simulink model "chap6_6sim"  (Simulink 6.3)
settings: Solver=ode45  StartTime=0.0  StopTime=10  FixedStep=0.001  RelTol=1e-3
settings Model: Creator=hp  LastModifiedBy=Administrator
settings DebuggingCC: SolverPrmCheckMsg=none

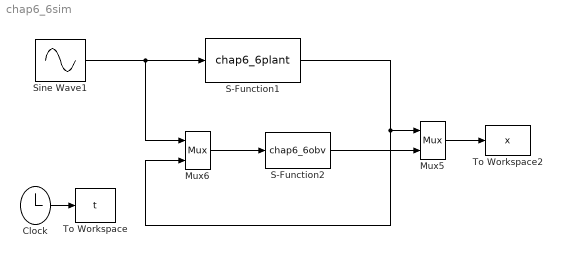
== system chap6_6sim ==
  Clock : Clock
      settings: Decimation=30
  Mux5 : Mux  Inputs=2
  Mux6 : Mux  Inputs=2
  S-Function1 : S-Function  FunctionName=chap6_6plant
  S-Function2 : S-Function  FunctionName=chap6_6obv
  Sine Wave1 : Sin  SampleTime=0
  To Workspace : ToWorkspace  VariableName=t  SampleTime=-1  SaveFormat=Array
  To Workspace2 : ToWorkspace  VariableName=x  SampleTime=-1  SaveFormat=Array
  wires:
  Mux6/1 -> S-Function2/1
  Clock/1 -> To Workspace/1
  S-Function1/1 -> Mux5/1, Mux6/2
  S-Function2/1 -> Mux5/2
  Mux5/1 -> To Workspace2/1
  Sine Wave1/1 -> S-Function1/1, Mux6/1
